simulink model "NUgus_IK"  (R2018a)
settings: Solver=VariableStepAuto  StartTime=0.0  StopTime=inf  RelTol=1e-3
values from neighbouring files (symbols this model uses):
  CM740_acc_bias = 4 * 9.80743    (= 39.22972)    [CM740_init.m]
  CM740_acc_gain = 512 / CM740_acc_centre    [CM740_init.m]
  CM740_gyro_bias = 1600 / 360 * 2 * pi    (= 27.9252680319)    [CM740_init.m]
  CM740_gyro_gain = 512 / CM740_gyro_centre    [CM740_init.m]
  head = [-0.05482228998067195, -0.00010888238321339966, 0.0011712900228573724, 0.41900000000000004]    [comtest.m]
  s = mean(abs(present_speed.data))    [RunServoTest.m]
  torso = [0.0050079703254699804, 0.008880921777563762, 0.1021503146237477, 2.5390000000000006]    [comtest.m]
undefined symbols (not defined in the file or in its folder): floor, X, Y, Z
libraries: sm_lib x211, fl_lib x128, nesl_utility x68
(part 7 of 8)

== system NUgus_IK/NUgus/right_foot/foot_bl_contact ==
  6-DOF Joint : sm_lib/Joints/6-DOF Joint  SenseConstraintForce=off  SenseConstraintForceX=off  SenseConstraintForceY=off  SenseConstraintForceZ=off  SenseConstraintTorque=off  SenseConstraintTorqueX=off  SenseConstraintTorqueY=off  SenseConstraintTorqueZ=off  SenseTotalForce=off  SenseTotalForceX=off  SenseTotalForceY=off  SenseTotalForceZ=off  SenseTotalTorque=off  SenseTotalTorqueX=off  SenseTotalTorqueY=off  SenseTotalTorqueZ=off  CompositeWrenchDir=FollowerOnBase  CompositeWrenchFrame=BaseFrame  PxEquilibriumPosition=0  PxEquilibriumPositionUnits=m  PxSpringStiffness=0  PxSpringStiffnessUnits=N/m  PxDampingCoefficient=0  PxDampingCoefficientUnits=N/(m/s)  PxTorqueActuationMode=InputTorque  PxMotionActuationMode=ComputedMotion  PxSensePosition=off  PxSenseVelocity=on  PxSenseAcceleration=off  PxSenseTorqueForce=off  PxPositionTargetSpecify=off  PxPositionTargetPriority=High  PxPositionTargetValue=0  PxPositionTargetValueUnits=m  PxVelocityTargetSpecify=off  PxVelocityTargetPriority=High  PxVelocityTargetValue=0  PxVelocityTargetValueUnits=m/s  PyEquilibriumPosition=0  PyEquilibriumPositionUnits=m  PySpringStiffness=0  PySpringStiffnessUnits=N/m  PyDampingCoefficient=0  PyDampingCoefficientUnits=N/(m/s)  PyTorqueActuationMode=InputTorque  PyMotionActuationMode=ComputedMotion  PySensePosition=off  PySenseVelocity=on  PySenseAcceleration=off  PySenseTorqueForce=off  PyPositionTargetSpecify=off  PyPositionTargetPriority=High  PyPositionTargetValue=0  PyPositionTargetValueUnits=m  PyVelocityTargetSpecify=off  PyVelocityTargetPriority=High  PyVelocityTargetValue=0  PyVelocityTargetValueUnits=m/s  PzEquilibriumPosition=0  PzEquilibriumPositionUnits=m  PzSpringStiffness=0  PzSpringStiffnessUnits=N/m  PzDampingCoefficient=0  PzDampingCoefficientUnits=N/(m/s)  PzTorqueActuationMode=InputTorque  PzMotionActuationMode=ComputedMotion  PzSensePosition=on  PzSenseVelocity=on  PzSenseAcceleration=off  PzSenseTorqueForce=off  PzPositionTargetSpecify=off  PzPositionTargetPriority=High  PzPositionTargetValue=0  PzPositionTargetValueUnits=m  PzVelocityTargetSpecify=off  PzVelocityTargetPriority=High  PzVelocityTargetValue=0  PzVelocityTargetValueUnits=m/s  SphDefPosRotationMethod=None  SphDefPosRotationAngleUnits=deg  SphDefPosRotationStandardAxis=+Z  SphDefPosRotationAngle=0.0  SphDefPosRotationArbitraryAxis=[0 0 1]  SphDefPosFollAlignAxisA=+X  SphDefPosBaseAlignAxisA=+Y  SphDefPosFollAlignAxisB=+Y  SphDefPosBaseAlignAxisB=+Z  SphDefPosRotationSequenceAxes=FollowerAxes  SphDefPosRotationSequence=XYX  SphDefPosRotationSequenceAngles=[0 0 0]  SphDefPosRotationSequenceAnglesUnits=deg  SphDefPosRotationMatrix=[1 0 0; 0 1 0; 0 0 1]  SphEqPosRotationMethod=None  SphEqPosRotationAngleUnits=deg  SphEqPosRotationStandardAxis=+Z  SphEqPosRotationAngle=0.0  SphEqPosRotationArbitraryAxis=[0 0 1]  SphEqPosFollAlignAxisA=+X  SphEqPosBaseAlignAxisA=+Y  SphEqPosFollAlignAxisB=+Y  SphEqPosBaseAlignAxisB=+Z  SphEqPosRotationSequenceAxes=FollowerAxes  SphEqPosRotationSequence=XYX  SphEqPosRotationSequenceAngles=[0 0 0]  SphEqPosRotationSequenceAnglesUnits=deg  SphEqPosRotationMatrix=[1 0 0; 0 1 0; 0 0 1]  SphSpringStiffness=0  SphSpringStiffnessUnits=N*m/deg  SphDampingCoefficient=0  SphDampingCoefficientUnits=N*m/(deg/s)  SphActuateTorqueX=off  SphActuateTorqueY=off  SphActuateTorqueZ=off  SphActuateTorque=off  SphTorqueActuationMode=NoTorque  SphMotionActuationMode=ComputedMotion  SphActuationFrame=BaseFrame  SphSensePosition=off  SphSenseVelocityX=off  SphSenseVelocityY=off  SphSenseVelocityZ=off  SphSenseVelocity=off  SphSenseAccelerationX=off  SphSenseAccelerationY=off  SphSenseAccelerationZ=off  SphSenseAcceleration=off  SphSenseTorqueX=off  SphSenseTorqueY=off  SphSenseTorqueZ=off  SphSenseTorqueForce=off  SphSensingFrame=BaseFrame  SphPositionTargetRotationMethod=None  SphPositionTargetRotationAngleUnits=deg  SphPositionTargetRotationStandardAxis=+Z  SphPositionTargetRotationAngle=0.0  SphPositionTargetRotationArbitraryAxis=[0 0 1]  SphPositionTargetFollAlignAxisA=+X  SphPositionTargetBaseAlignAxisA=+Y  SphPositionTargetFollAlignAxisB=+Y  SphPositionTargetBaseAlignAxisB=+Z  SphPositionTargetRotationSequenceAxes=FollowerAxes  SphPositionTargetRotationSequence=XYX  SphPositionTargetRotationSequenceAngles=[0 0 0]  SphPositionTargetRotationSequenceAnglesUnits=deg  SphPositionTargetRotationMatrix=[1 0 0; 0 1 0; 0 0 1]  SphPositionTargetSpecify=off  SphPositionTargetPriority=High  SphVelocityTargetValue=[0 0 0]  SphVelocityTargetValueUnits=deg/s  SphVelocityTargetSpecify=off  SphVelocityTargetPriority=High  SphVelocityTargetInFollowerFrame=on
  PS Abs1 : fl_lib/Physical Signals/Nonlinear Operators/PS Abs
      settings: SourceProductName=Simscape  SourceProductBaseCode=SS
  PS Add : fl_lib/Physical Signals/Functions/PS Add
  PS Gain : fl_lib/Physical Signals/Functions/PS Gain  gain=floor.friction
  calculate forces : Subsystem
  x Velocity Gain : fl_lib/Physical Signals/Functions/PS Gain  gain=floor.vel_gain
  y Velocity Gain : fl_lib/Physical Signals/Functions/PS Gain  gain=floor.vel_gain
  z Position Gain : fl_lib/Physical Signals/Functions/PS Gain  gain=floor.pos_gain
  z Velocity Gain : fl_lib/Physical Signals/Functions/PS Gain  gain=floor.vel_gain
  Contact : PMIOPort  Side=Right
  Floor : PMIOPort  Port=2  Side=Left
  connections:
  6-DOF Joint/RConn1 -- Contact/RConn1
  Floor/RConn1 -- 6-DOF Joint/LConn1
  6-DOF Joint/RConn4 -- calculate forces/LConn3 -- z Position Gain/LConn1
  z Velocity Gain/LConn1 -- 6-DOF Joint/RConn5
  y Velocity Gain/LConn1 -- 6-DOF Joint/RConn3
  x Velocity Gain/LConn1 -- 6-DOF Joint/RConn2
  PS Add/LConn1 -- z Position Gain/RConn1
  PS Add/LConn2 -- z Velocity Gain/RConn1
  PS Abs1/LConn1 -- PS Gain/RConn1
  PS Add/RConn1 -- calculate forces/LConn4 -- PS Gain/LConn1
  x Velocity Gain/RConn1 -- calculate forces/LConn1
  y Velocity Gain/RConn1 -- calculate forces/LConn2
  PS Abs1/RConn1 -- calculate forces/LConn5
  calculate forces/RConn1 -- 6-DOF Joint/LConn2
  calculate forces/RConn2 -- 6-DOF Joint/LConn3
  calculate forces/RConn3 -- 6-DOF Joint/LConn4

== system NUgus_IK/NUgus/right_foot/foot_br_contact ==
  6-DOF Joint : sm_lib/Joints/6-DOF Joint  SenseConstraintForce=off  SenseConstraintForceX=off  SenseConstraintForceY=off  SenseConstraintForceZ=off  SenseConstraintTorque=off  SenseConstraintTorqueX=off  SenseConstraintTorqueY=off  SenseConstraintTorqueZ=off  SenseTotalForce=off  SenseTotalForceX=off  SenseTotalForceY=off  SenseTotalForceZ=off  SenseTotalTorque=off  SenseTotalTorqueX=off  SenseTotalTorqueY=off  SenseTotalTorqueZ=off  CompositeWrenchDir=FollowerOnBase  CompositeWrenchFrame=BaseFrame  PxEquilibriumPosition=0  PxEquilibriumPositionUnits=m  PxSpringStiffness=0  PxSpringStiffnessUnits=N/m  PxDampingCoefficient=0  PxDampingCoefficientUnits=N/(m/s)  PxTorqueActuationMode=InputTorque  PxMotionActuationMode=ComputedMotion  PxSensePosition=off  PxSenseVelocity=on  PxSenseAcceleration=off  PxSenseTorqueForce=off  PxPositionTargetSpecify=off  PxPositionTargetPriority=High  PxPositionTargetValue=0  PxPositionTargetValueUnits=m  PxVelocityTargetSpecify=off  PxVelocityTargetPriority=High  PxVelocityTargetValue=0  PxVelocityTargetValueUnits=m/s  PyEquilibriumPosition=0  PyEquilibriumPositionUnits=m  PySpringStiffness=0  PySpringStiffnessUnits=N/m  PyDampingCoefficient=0  PyDampingCoefficientUnits=N/(m/s)  PyTorqueActuationMode=InputTorque  PyMotionActuationMode=ComputedMotion  PySensePosition=off  PySenseVelocity=on  PySenseAcceleration=off  PySenseTorqueForce=off  PyPositionTargetSpecify=off  PyPositionTargetPriority=High  PyPositionTargetValue=0  PyPositionTargetValueUnits=m  PyVelocityTargetSpecify=off  PyVelocityTargetPriority=High  PyVelocityTargetValue=0  PyVelocityTargetValueUnits=m/s  PzEquilibriumPosition=0  PzEquilibriumPositionUnits=m  PzSpringStiffness=0  PzSpringStiffnessUnits=N/m  PzDampingCoefficient=0  PzDampingCoefficientUnits=N/(m/s)  PzTorqueActuationMode=InputTorque  PzMotionActuationMode=ComputedMotion  PzSensePosition=on  PzSenseVelocity=on  PzSenseAcceleration=off  PzSenseTorqueForce=off  PzPositionTargetSpecify=off  PzPositionTargetPriority=High  PzPositionTargetValue=0  PzPositionTargetValueUnits=m  PzVelocityTargetSpecify=off  PzVelocityTargetPriority=High  PzVelocityTargetValue=0  PzVelocityTargetValueUnits=m/s  SphDefPosRotationMethod=None  SphDefPosRotationAngleUnits=deg  SphDefPosRotationStandardAxis=+Z  SphDefPosRotationAngle=0.0  SphDefPosRotationArbitraryAxis=[0 0 1]  SphDefPosFollAlignAxisA=+X  SphDefPosBaseAlignAxisA=+Y  SphDefPosFollAlignAxisB=+Y  SphDefPosBaseAlignAxisB=+Z  SphDefPosRotationSequenceAxes=FollowerAxes  SphDefPosRotationSequence=XYX  SphDefPosRotationSequenceAngles=[0 0 0]  SphDefPosRotationSequenceAnglesUnits=deg  SphDefPosRotationMatrix=[1 0 0; 0 1 0; 0 0 1]  SphEqPosRotationMethod=None  SphEqPosRotationAngleUnits=deg  SphEqPosRotationStandardAxis=+Z  SphEqPosRotationAngle=0.0  SphEqPosRotationArbitraryAxis=[0 0 1]  SphEqPosFollAlignAxisA=+X  SphEqPosBaseAlignAxisA=+Y  SphEqPosFollAlignAxisB=+Y  SphEqPosBaseAlignAxisB=+Z  SphEqPosRotationSequenceAxes=FollowerAxes  SphEqPosRotationSequence=XYX  SphEqPosRotationSequenceAngles=[0 0 0]  SphEqPosRotationSequenceAnglesUnits=deg  SphEqPosRotationMatrix=[1 0 0; 0 1 0; 0 0 1]  SphSpringStiffness=0  SphSpringStiffnessUnits=N*m/deg  SphDampingCoefficient=0  SphDampingCoefficientUnits=N*m/(deg/s)  SphActuateTorqueX=off  SphActuateTorqueY=off  SphActuateTorqueZ=off  SphActuateTorque=off  SphTorqueActuationMode=NoTorque  SphMotionActuationMode=ComputedMotion  SphActuationFrame=BaseFrame  SphSensePosition=off  SphSenseVelocityX=off  SphSenseVelocityY=off  SphSenseVelocityZ=off  SphSenseVelocity=off  SphSenseAccelerationX=off  SphSenseAccelerationY=off  SphSenseAccelerationZ=off  SphSenseAcceleration=off  SphSenseTorqueX=off  SphSenseTorqueY=off  SphSenseTorqueZ=off  SphSenseTorqueForce=off  SphSensingFrame=BaseFrame  SphPositionTargetRotationMethod=None  SphPositionTargetRotationAngleUnits=deg  SphPositionTargetRotationStandardAxis=+Z  SphPositionTargetRotationAngle=0.0  SphPositionTargetRotationArbitraryAxis=[0 0 1]  SphPositionTargetFollAlignAxisA=+X  SphPositionTargetBaseAlignAxisA=+Y  SphPositionTargetFollAlignAxisB=+Y  SphPositionTargetBaseAlignAxisB=+Z  SphPositionTargetRotationSequenceAxes=FollowerAxes  SphPositionTargetRotationSequence=XYX  SphPositionTargetRotationSequenceAngles=[0 0 0]  SphPositionTargetRotationSequenceAnglesUnits=deg  SphPositionTargetRotationMatrix=[1 0 0; 0 1 0; 0 0 1]  SphPositionTargetSpecify=off  SphPositionTargetPriority=High  SphVelocityTargetValue=[0 0 0]  SphVelocityTargetValueUnits=deg/s  SphVelocityTargetSpecify=off  SphVelocityTargetPriority=High  SphVelocityTargetInFollowerFrame=on
  PS Abs1 : fl_lib/Physical Signals/Nonlinear Operators/PS Abs
      settings: SourceProductName=Simscape  SourceProductBaseCode=SS
  PS Add : fl_lib/Physical Signals/Functions/PS Add
  PS Gain : fl_lib/Physical Signals/Functions/PS Gain  gain=floor.friction
  calculate forces : Subsystem
  x Velocity Gain : fl_lib/Physical Signals/Functions/PS Gain  gain=floor.vel_gain
  y Velocity Gain : fl_lib/Physical Signals/Functions/PS Gain  gain=floor.vel_gain
  z Position Gain : fl_lib/Physical Signals/Functions/PS Gain  gain=floor.pos_gain
  z Velocity Gain : fl_lib/Physical Signals/Functions/PS Gain  gain=floor.vel_gain
  Contact : PMIOPort  Side=Right
  Floor : PMIOPort  Port=2  Side=Left
  connections:
  6-DOF Joint/RConn1 -- Contact/RConn1
  Floor/RConn1 -- 6-DOF Joint/LConn1
  6-DOF Joint/RConn4 -- calculate forces/LConn3 -- z Position Gain/LConn1
  z Velocity Gain/LConn1 -- 6-DOF Joint/RConn5
  y Velocity Gain/LConn1 -- 6-DOF Joint/RConn3
  x Velocity Gain/LConn1 -- 6-DOF Joint/RConn2
  PS Add/LConn1 -- z Position Gain/RConn1
  PS Add/LConn2 -- z Velocity Gain/RConn1
  PS Abs1/LConn1 -- PS Gain/RConn1
  PS Add/RConn1 -- calculate forces/LConn4 -- PS Gain/LConn1
  x Velocity Gain/RConn1 -- calculate forces/LConn1
  y Velocity Gain/RConn1 -- calculate forces/LConn2
  PS Abs1/RConn1 -- calculate forces/LConn5
  calculate forces/RConn1 -- 6-DOF Joint/LConn2
  calculate forces/RConn2 -- 6-DOF Joint/LConn3
  calculate forces/RConn3 -- 6-DOF Joint/LConn4

== system NUgus_IK/NUgus/right_foot/foot_fl_contact ==
  6-DOF Joint : sm_lib/Joints/6-DOF Joint  SenseConstraintForce=off  SenseConstraintForceX=off  SenseConstraintForceY=off  SenseConstraintForceZ=off  SenseConstraintTorque=off  SenseConstraintTorqueX=off  SenseConstraintTorqueY=off  SenseConstraintTorqueZ=off  SenseTotalForce=off  SenseTotalForceX=off  SenseTotalForceY=off  SenseTotalForceZ=off  SenseTotalTorque=off  SenseTotalTorqueX=off  SenseTotalTorqueY=off  SenseTotalTorqueZ=off  CompositeWrenchDir=FollowerOnBase  CompositeWrenchFrame=BaseFrame  PxEquilibriumPosition=0  PxEquilibriumPositionUnits=m  PxSpringStiffness=0  PxSpringStiffnessUnits=N/m  PxDampingCoefficient=0  PxDampingCoefficientUnits=N/(m/s)  PxTorqueActuationMode=InputTorque  PxMotionActuationMode=ComputedMotion  PxSensePosition=off  PxSenseVelocity=on  PxSenseAcceleration=off  PxSenseTorqueForce=off  PxPositionTargetSpecify=off  PxPositionTargetPriority=High  PxPositionTargetValue=0  PxPositionTargetValueUnits=m  PxVelocityTargetSpecify=off  PxVelocityTargetPriority=High  PxVelocityTargetValue=0  PxVelocityTargetValueUnits=m/s  PyEquilibriumPosition=0  PyEquilibriumPositionUnits=m  PySpringStiffness=0  PySpringStiffnessUnits=N/m  PyDampingCoefficient=0  PyDampingCoefficientUnits=N/(m/s)  PyTorqueActuationMode=InputTorque  PyMotionActuationMode=ComputedMotion  PySensePosition=off  PySenseVelocity=on  PySenseAcceleration=off  PySenseTorqueForce=off  PyPositionTargetSpecify=off  PyPositionTargetPriority=High  PyPositionTargetValue=0  PyPositionTargetValueUnits=m  PyVelocityTargetSpecify=off  PyVelocityTargetPriority=High  PyVelocityTargetValue=0  PyVelocityTargetValueUnits=m/s  PzEquilibriumPosition=0  PzEquilibriumPositionUnits=m  PzSpringStiffness=0  PzSpringStiffnessUnits=N/m  PzDampingCoefficient=0  PzDampingCoefficientUnits=N/(m/s)  PzTorqueActuationMode=InputTorque  PzMotionActuationMode=ComputedMotion  PzSensePosition=on  PzSenseVelocity=on  PzSenseAcceleration=off  PzSenseTorqueForce=off  PzPositionTargetSpecify=off  PzPositionTargetPriority=High  PzPositionTargetValue=0  PzPositionTargetValueUnits=m  PzVelocityTargetSpecify=off  PzVelocityTargetPriority=High  PzVelocityTargetValue=0  PzVelocityTargetValueUnits=m/s  SphDefPosRotationMethod=None  SphDefPosRotationAngleUnits=deg  SphDefPosRotationStandardAxis=+Z  SphDefPosRotationAngle=0.0  SphDefPosRotationArbitraryAxis=[0 0 1]  SphDefPosFollAlignAxisA=+X  SphDefPosBaseAlignAxisA=+Y  SphDefPosFollAlignAxisB=+Y  SphDefPosBaseAlignAxisB=+Z  SphDefPosRotationSequenceAxes=FollowerAxes  SphDefPosRotationSequence=XYX  SphDefPosRotationSequenceAngles=[0 0 0]  SphDefPosRotationSequenceAnglesUnits=deg  SphDefPosRotationMatrix=[1 0 0; 0 1 0; 0 0 1]  SphEqPosRotationMethod=None  SphEqPosRotationAngleUnits=deg  SphEqPosRotationStandardAxis=+Z  SphEqPosRotationAngle=0.0  SphEqPosRotationArbitraryAxis=[0 0 1]  SphEqPosFollAlignAxisA=+X  SphEqPosBaseAlignAxisA=+Y  SphEqPosFollAlignAxisB=+Y  SphEqPosBaseAlignAxisB=+Z  SphEqPosRotationSequenceAxes=FollowerAxes  SphEqPosRotationSequence=XYX  SphEqPosRotationSequenceAngles=[0 0 0]  SphEqPosRotationSequenceAnglesUnits=deg  SphEqPosRotationMatrix=[1 0 0; 0 1 0; 0 0 1]  SphSpringStiffness=0  SphSpringStiffnessUnits=N*m/deg  SphDampingCoefficient=0  SphDampingCoefficientUnits=N*m/(deg/s)  SphActuateTorqueX=off  SphActuateTorqueY=off  SphActuateTorqueZ=off  SphActuateTorque=off  SphTorqueActuationMode=NoTorque  SphMotionActuationMode=ComputedMotion  SphActuationFrame=BaseFrame  SphSensePosition=off  SphSenseVelocityX=off  SphSenseVelocityY=off  SphSenseVelocityZ=off  SphSenseVelocity=off  SphSenseAccelerationX=off  SphSenseAccelerationY=off  SphSenseAccelerationZ=off  SphSenseAcceleration=off  SphSenseTorqueX=off  SphSenseTorqueY=off  SphSenseTorqueZ=off  SphSenseTorqueForce=off  SphSensingFrame=BaseFrame  SphPositionTargetRotationMethod=None  SphPositionTargetRotationAngleUnits=deg  SphPositionTargetRotationStandardAxis=+Z  SphPositionTargetRotationAngle=0.0  SphPositionTargetRotationArbitraryAxis=[0 0 1]  SphPositionTargetFollAlignAxisA=+X  SphPositionTargetBaseAlignAxisA=+Y  SphPositionTargetFollAlignAxisB=+Y  SphPositionTargetBaseAlignAxisB=+Z  SphPositionTargetRotationSequenceAxes=FollowerAxes  SphPositionTargetRotationSequence=XYX  SphPositionTargetRotationSequenceAngles=[0 0 0]  SphPositionTargetRotationSequenceAnglesUnits=deg  SphPositionTargetRotationMatrix=[1 0 0; 0 1 0; 0 0 1]  SphPositionTargetSpecify=off  SphPositionTargetPriority=High  SphVelocityTargetValue=[0 0 0]  SphVelocityTargetValueUnits=deg/s  SphVelocityTargetSpecify=off  SphVelocityTargetPriority=High  SphVelocityTargetInFollowerFrame=on
  PS Abs1 : fl_lib/Physical Signals/Nonlinear Operators/PS Abs
      settings: SourceProductName=Simscape  SourceProductBaseCode=SS
  PS Add : fl_lib/Physical Signals/Functions/PS Add
  PS Gain : fl_lib/Physical Signals/Functions/PS Gain  gain=floor.friction
  calculate forces : Subsystem
  x Velocity Gain : fl_lib/Physical Signals/Functions/PS Gain  gain=floor.vel_gain
  y Velocity Gain : fl_lib/Physical Signals/Functions/PS Gain  gain=floor.vel_gain
  z Position Gain : fl_lib/Physical Signals/Functions/PS Gain  gain=floor.pos_gain
  z Velocity Gain : fl_lib/Physical Signals/Functions/PS Gain  gain=floor.vel_gain
  Contact : PMIOPort  Side=Right
  Floor : PMIOPort  Port=2  Side=Left
  connections:
  6-DOF Joint/RConn1 -- Contact/RConn1
  Floor/RConn1 -- 6-DOF Joint/LConn1
  6-DOF Joint/RConn4 -- calculate forces/LConn3 -- z Position Gain/LConn1
  z Velocity Gain/LConn1 -- 6-DOF Joint/RConn5
  y Velocity Gain/LConn1 -- 6-DOF Joint/RConn3
  x Velocity Gain/LConn1 -- 6-DOF Joint/RConn2
  PS Add/LConn1 -- z Position Gain/RConn1
  PS Add/LConn2 -- z Velocity Gain/RConn1
  PS Abs1/LConn1 -- PS Gain/RConn1
  PS Add/RConn1 -- calculate forces/LConn4 -- PS Gain/LConn1
  x Velocity Gain/RConn1 -- calculate forces/LConn1
  y Velocity Gain/RConn1 -- calculate forces/LConn2
  PS Abs1/RConn1 -- calculate forces/LConn5
  calculate forces/RConn1 -- 6-DOF Joint/LConn2
  calculate forces/RConn2 -- 6-DOF Joint/LConn3
  calculate forces/RConn3 -- 6-DOF Joint/LConn4

== system NUgus_IK/NUgus/right_foot/foot_fr_contact ==
  6-DOF Joint : sm_lib/Joints/6-DOF Joint  SenseConstraintForce=off  SenseConstraintForceX=off  SenseConstraintForceY=off  SenseConstraintForceZ=off  SenseConstraintTorque=off  SenseConstraintTorqueX=off  SenseConstraintTorqueY=off  SenseConstraintTorqueZ=off  SenseTotalForce=off  SenseTotalForceX=off  SenseTotalForceY=off  SenseTotalForceZ=off  SenseTotalTorque=off  SenseTotalTorqueX=off  SenseTotalTorqueY=off  SenseTotalTorqueZ=off  CompositeWrenchDir=FollowerOnBase  CompositeWrenchFrame=BaseFrame  PxEquilibriumPosition=0  PxEquilibriumPositionUnits=m  PxSpringStiffness=0  PxSpringStiffnessUnits=N/m  PxDampingCoefficient=0  PxDampingCoefficientUnits=N/(m/s)  PxTorqueActuationMode=InputTorque  PxMotionActuationMode=ComputedMotion  PxSensePosition=off  PxSenseVelocity=on  PxSenseAcceleration=off  PxSenseTorqueForce=off  PxPositionTargetSpecify=off  PxPositionTargetPriority=High  PxPositionTargetValue=0  PxPositionTargetValueUnits=m  PxVelocityTargetSpecify=off  PxVelocityTargetPriority=High  PxVelocityTargetValue=0  PxVelocityTargetValueUnits=m/s  PyEquilibriumPosition=0  PyEquilibriumPositionUnits=m  PySpringStiffness=0  PySpringStiffnessUnits=N/m  PyDampingCoefficient=0  PyDampingCoefficientUnits=N/(m/s)  PyTorqueActuationMode=InputTorque  PyMotionActuationMode=ComputedMotion  PySensePosition=off  PySenseVelocity=on  PySenseAcceleration=off  PySenseTorqueForce=off  PyPositionTargetSpecify=off  PyPositionTargetPriority=High  PyPositionTargetValue=0  PyPositionTargetValueUnits=m  PyVelocityTargetSpecify=off  PyVelocityTargetPriority=High  PyVelocityTargetValue=0  PyVelocityTargetValueUnits=m/s  PzEquilibriumPosition=0  PzEquilibriumPositionUnits=m  PzSpringStiffness=0  PzSpringStiffnessUnits=N/m  PzDampingCoefficient=0  PzDampingCoefficientUnits=N/(m/s)  PzTorqueActuationMode=InputTorque  PzMotionActuationMode=ComputedMotion  PzSensePosition=on  PzSenseVelocity=on  PzSenseAcceleration=off  PzSenseTorqueForce=off  PzPositionTargetSpecify=off  PzPositionTargetPriority=High  PzPositionTargetValue=0  PzPositionTargetValueUnits=m  PzVelocityTargetSpecify=off  PzVelocityTargetPriority=High  PzVelocityTargetValue=0  PzVelocityTargetValueUnits=m/s  SphDefPosRotationMethod=None  SphDefPosRotationAngleUnits=deg  SphDefPosRotationStandardAxis=+Z  SphDefPosRotationAngle=0.0  SphDefPosRotationArbitraryAxis=[0 0 1]  SphDefPosFollAlignAxisA=+X  SphDefPosBaseAlignAxisA=+Y  SphDefPosFollAlignAxisB=+Y  SphDefPosBaseAlignAxisB=+Z  SphDefPosRotationSequenceAxes=FollowerAxes  SphDefPosRotationSequence=XYX  SphDefPosRotationSequenceAngles=[0 0 0]  SphDefPosRotationSequenceAnglesUnits=deg  SphDefPosRotationMatrix=[1 0 0; 0 1 0; 0 0 1]  SphEqPosRotationMethod=None  SphEqPosRotationAngleUnits=deg  SphEqPosRotationStandardAxis=+Z  SphEqPosRotationAngle=0.0  SphEqPosRotationArbitraryAxis=[0 0 1]  SphEqPosFollAlignAxisA=+X  SphEqPosBaseAlignAxisA=+Y  SphEqPosFollAlignAxisB=+Y  SphEqPosBaseAlignAxisB=+Z  SphEqPosRotationSequenceAxes=FollowerAxes  SphEqPosRotationSequence=XYX  SphEqPosRotationSequenceAngles=[0 0 0]  SphEqPosRotationSequenceAnglesUnits=deg  SphEqPosRotationMatrix=[1 0 0; 0 1 0; 0 0 1]  SphSpringStiffness=0  SphSpringStiffnessUnits=N*m/deg  SphDampingCoefficient=0  SphDampingCoefficientUnits=N*m/(deg/s)  SphActuateTorqueX=off  SphActuateTorqueY=off  SphActuateTorqueZ=off  SphActuateTorque=off  SphTorqueActuationMode=NoTorque  SphMotionActuationMode=ComputedMotion  SphActuationFrame=BaseFrame  SphSensePosition=off  SphSenseVelocityX=off  SphSenseVelocityY=off  SphSenseVelocityZ=off  SphSenseVelocity=off  SphSenseAccelerationX=off  SphSenseAccelerationY=off  SphSenseAccelerationZ=off  SphSenseAcceleration=off  SphSenseTorqueX=off  SphSenseTorqueY=off  SphSenseTorqueZ=off  SphSenseTorqueForce=off  SphSensingFrame=BaseFrame  SphPositionTargetRotationMethod=None  SphPositionTargetRotationAngleUnits=deg  SphPositionTargetRotationStandardAxis=+Z  SphPositionTargetRotationAngle=0.0  SphPositionTargetRotationArbitraryAxis=[0 0 1]  SphPositionTargetFollAlignAxisA=+X  SphPositionTargetBaseAlignAxisA=+Y  SphPositionTargetFollAlignAxisB=+Y  SphPositionTargetBaseAlignAxisB=+Z  SphPositionTargetRotationSequenceAxes=FollowerAxes  SphPositionTargetRotationSequence=XYX  SphPositionTargetRotationSequenceAngles=[0 0 0]  SphPositionTargetRotationSequenceAnglesUnits=deg  SphPositionTargetRotationMatrix=[1 0 0; 0 1 0; 0 0 1]  SphPositionTargetSpecify=off  SphPositionTargetPriority=High  SphVelocityTargetValue=[0 0 0]  SphVelocityTargetValueUnits=deg/s  SphVelocityTargetSpecify=off  SphVelocityTargetPriority=High  SphVelocityTargetInFollowerFrame=on
  PS Abs1 : fl_lib/Physical Signals/Nonlinear Operators/PS Abs
      settings: SourceProductName=Simscape  SourceProductBaseCode=SS
  PS Add : fl_lib/Physical Signals/Functions/PS Add
  PS Gain : fl_lib/Physical Signals/Functions/PS Gain  gain=floor.friction
  calculate forces : Subsystem
  x Velocity Gain : fl_lib/Physical Signals/Functions/PS Gain  gain=floor.vel_gain
  y Velocity Gain : fl_lib/Physical Signals/Functions/PS Gain  gain=floor.vel_gain
  z Position Gain : fl_lib/Physical Signals/Functions/PS Gain  gain=floor.pos_gain
  z Velocity Gain : fl_lib/Physical Signals/Functions/PS Gain  gain=floor.vel_gain
  Contact : PMIOPort  Side=Right
  Floor : PMIOPort  Port=2  Side=Left
  connections:
  6-DOF Joint/RConn1 -- Contact/RConn1
  Floor/RConn1 -- 6-DOF Joint/LConn1
  6-DOF Joint/RConn4 -- calculate forces/LConn3 -- z Position Gain/LConn1
  z Velocity Gain/LConn1 -- 6-DOF Joint/RConn5
  y Velocity Gain/LConn1 -- 6-DOF Joint/RConn3
  x Velocity Gain/LConn1 -- 6-DOF Joint/RConn2
  PS Add/LConn1 -- z Position Gain/RConn1
  PS Add/LConn2 -- z Velocity Gain/RConn1
  PS Abs1/LConn1 -- PS Gain/RConn1
  PS Add/RConn1 -- calculate forces/LConn4 -- PS Gain/LConn1
  x Velocity Gain/RConn1 -- calculate forces/LConn1
  y Velocity Gain/RConn1 -- calculate forces/LConn2
  PS Abs1/RConn1 -- calculate forces/LConn5
  calculate forces/RConn1 -- 6-DOF Joint/LConn2
  calculate forces/RConn2 -- 6-DOF Joint/LConn3
  calculate forces/RConn3 -- 6-DOF Joint/LConn4

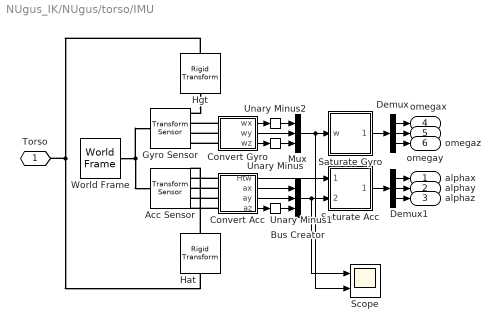
== system NUgus_IK/NUgus/torso/IMU ==
  Acc Sensor : sm_lib/Frames and Transforms/Transform Sensor  MeasurementFrame=Follower  SenseAngle=off  SenseAxis=off  SenseAngle1=off  SenseAngle2=off  SenseAngle3=off  SenseQ=off  SenseR=on  SenseOmegaX=off  SenseOmegaY=off  SenseOmegaZ=off  SenseOmega1=off  SenseOmega2=off  SenseOmega3=off  SenseQDot=off  SenseRDot=off  SenseAlphaX=off  SenseAlphaY=off  SenseAlphaZ=off  SenseAlpha1=off  SenseAlpha2=off  SenseAlpha3=off  SenseQDDot=off  SenseRDDot=off  SenseX=off  SenseY=off  SenseZ=off  SenseRad=off  SenseAzim=off  SenseDist=off  SenseInc=off  SenseXDot=off  SenseYDot=off  SenseZDot=off  SenseRadDot=off  SenseAzimDot=off  SenseDistDot=off  SenseIncDot=off  SenseXDDot=on  SenseYDDot=on  SenseZDDot=on  SenseRadDDot=off  SenseAzimDDot=off  SenseDistDDot=off  SenseIncDDot=off
  Bus Creator : BusCreator  Inputs=3
  Convert Acc : Subsystem
  Convert Gyro : Subsystem
  Demux : Demux  Outputs=3
  Demux1 : Demux  Outputs=3
  Gyro Sensor : sm_lib/Frames and Transforms/Transform Sensor  MeasurementFrame=Follower  SenseAngle=off  SenseAxis=off  SenseAngle1=off  SenseAngle2=off  SenseAngle3=off  SenseQ=off  SenseR=off  SenseOmegaX=on  SenseOmegaY=on  SenseOmegaZ=on  SenseOmega1=off  SenseOmega2=off  SenseOmega3=off  SenseQDot=off  SenseRDot=off  SenseAlphaX=off  SenseAlphaY=off  SenseAlphaZ=off  SenseAlpha1=off  SenseAlpha2=off  SenseAlpha3=off  SenseQDDot=off  SenseRDDot=off  SenseX=off  SenseY=off  SenseZ=off  SenseRad=off  SenseAzim=off  SenseDist=off  SenseInc=off  SenseXDot=off  SenseYDot=off  SenseZDot=off  SenseRadDot=off  SenseAzimDot=off  SenseDistDot=off  SenseIncDot=off  SenseXDDot=off  SenseYDDot=off  SenseZDDot=off  SenseRadDDot=off  SenseAzimDDot=off  SenseDistDDot=off  SenseIncDDot=off
  Hat : sm_lib/Frames and Transforms/Rigid Transform  TranslationMethod=None  TranslationStandardOffset=0  TranslationLengthUnit=m  TranslationStandardAxis=+Z  TranslationCartesianOffset=[0 0 0]  TranslationROffset=0  TranslationROffsetUnits=m  TranslationZOffset=0  TranslationZOffsetUnits=m  TranslationThetaOffset=0  TranslationThetaOffsetUnits=deg  RotationMethod=None  RotationAngleUnits=deg  RotationStandardAxis=+Z  RotationAngle=0.0  RotationArbitraryAxis=[0 0 1]  FollAlignAxisA=+X  BaseAlignAxisA=+Y  FollAlignAxisB=+Y  BaseAlignAxisB=+Z  RotationSequenceAxes=FollowerAxes  RotationSequence=XYX  RotationSequenceAngles=[0 0 0]  RotationSequenceAnglesUnits=deg  RotationMatrix=[1 0 0; 0 1 0; 0 0 1]
  Hgt : sm_lib/Frames and Transforms/Rigid Transform  TranslationMethod=None  TranslationStandardOffset=0  TranslationLengthUnit=m  TranslationStandardAxis=+Z  TranslationCartesianOffset=[0 0 0]  TranslationROffset=0  TranslationROffsetUnits=m  TranslationZOffset=0  TranslationZOffsetUnits=m  TranslationThetaOffset=0  TranslationThetaOffsetUnits=deg  RotationMethod=None  RotationAngleUnits=deg  RotationStandardAxis=+Z  RotationAngle=0.0  RotationArbitraryAxis=[0 0 1]  FollAlignAxisA=+X  BaseAlignAxisA=+Y  FollAlignAxisB=+Y  BaseAlignAxisB=+Z  RotationSequenceAxes=FollowerAxes  RotationSequence=XYX  RotationSequenceAngles=[0 0 0]  RotationSequenceAnglesUnits=deg  RotationMatrix=[1 0 0; 0 1 0; 0 0 1]
  Mux : Mux  Inputs=3
  Saturate Acc : Subsystem
  Saturate Gyro : Subsystem
  Scope : Scope  NumInputPorts=2
  Unary Minus : UnaryMinus
  Unary Minus1 : UnaryMinus
  Unary Minus2 : UnaryMinus
  World Frame : sm_lib/Frames and Transforms/World Frame
  Torso : PMIOPort  Side=Left
  alphax : Outport
  alphay : Outport  Port=2
  alphaz : Outport  Port=3
  omegax : Outport  Port=4
  omegay : Outport  Port=5
  omegaz : Outport  Port=6
  wires:
  Convert Acc/3(ay) -> Bus Creator/2
  Convert Gyro/2(wy) -> Mux/2
  Convert Gyro/3(wz) -> Unary Minus/1
  Unary Minus/1 -> Mux/3
  Convert Gyro/1(wx) -> Unary Minus2/1
  Unary Minus2/1 -> Mux/1
  Convert Acc/2(ax) -> Bus Creator/1
  Unary Minus1/1 -> Bus Creator/3
  Demux/1 -> omegax/1
  Demux/2 -> omegay/1
  Demux/3 -> omegaz/1
  Demux1/3 -> alphaz/1
  Demux1/1 -> alphax/1
  Demux1/2 -> alphay/1
  Saturate Acc/1(alpha) -> Demux1/1
  Convert Acc/4(az) -> Unary Minus1/1
  Convert Acc/1(Htw) -> Saturate Acc/1(Hta)
  Bus Creator/1 -> Scope/1, Saturate Acc/2(Acc)
  Mux/1 -> Scope/2, Saturate Gyro/1(w)
  Saturate Gyro/1(omega) -> Demux/1
  connections:
  Convert Acc/LConn4 -- Acc Sensor/RConn5
  Convert Gyro/LConn2 -- Gyro Sensor/RConn3
  Convert Acc/LConn3 -- Acc Sensor/RConn4
  Hgt/LConn1 -- Hat/LConn1 -- Torso/RConn1
  Convert Gyro/LConn3 -- Gyro Sensor/RConn4
  Convert Acc/LConn2 -- Acc Sensor/RConn3
  Convert Gyro/LConn1 -- Gyro Sensor/RConn2
  World Frame/RConn1 -- Gyro Sensor/LConn1 -- Acc Sensor/LConn1
  Hat/RConn1 -- Acc Sensor/RConn1
  Convert Acc/LConn1 -- Acc Sensor/RConn2
  Hgt/RConn1 -- Gyro Sensor/RConn1

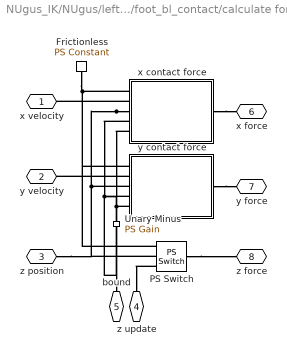
== system NUgus_IK/NUgus/left_foot/foot_bl_contact/calculate forces ==
  Frictionless : fl_lib/Physical Signals/Sources/PS Constant  constant=0
  PS Switch : fl_lib/Physical Signals/Nonlinear Operators/PS Switch  Threshold=0
      settings: SourceProductName=Simscape  SourceProductBaseCode=SS
  Unary Minus : fl_lib/Physical Signals/Functions/PS Gain  gain=-1
  x contact force : Subsystem
  y contact force : Subsystem
  x velocity : PMIOPort  Side=Left
  y velocity : PMIOPort  Port=2  Side=Left
  z position : PMIOPort  Port=3  Side=Left
  z update : PMIOPort  Port=4  Side=Left
  bound : PMIOPort  Port=5  Side=Left
  x force : PMIOPort  Port=6  Side=Right
  y force : PMIOPort  Port=7  Side=Right
  z force : PMIOPort  Port=8  Side=Right
  connections:
  x contact force/LConn2 -- x velocity/RConn1
  y contact force/LConn2 -- y velocity/RConn1
  y contact force/RConn1 -- y force/RConn1
  x contact force/RConn1 -- x force/RConn1
  PS Switch/RConn1 -- z force/RConn1
  x contact force/LConn3 -- PS Switch/LConn2 -- z position/RConn1 -- y contact force/LConn3
  x contact force/LConn4 -- Unary Minus/LConn1 -- bound/RConn1 -- y contact force/LConn4
  Unary Minus/RConn1 -- x contact force/LConn5 -- y contact force/LConn5
  x contact force/LConn1 -- y contact force/LConn1 -- PS Switch/LConn1 -- Frictionless/RConn1
  PS Switch/LConn3 -- z update/RConn1

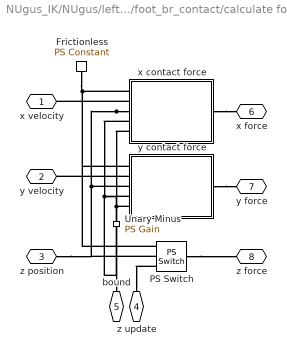
== system NUgus_IK/NUgus/left_foot/foot_br_contact/calculate forces ==
  Frictionless : fl_lib/Physical Signals/Sources/PS Constant  constant=0
  PS Switch : fl_lib/Physical Signals/Nonlinear Operators/PS Switch  Threshold=0
      settings: SourceProductName=Simscape  SourceProductBaseCode=SS
  Unary Minus : fl_lib/Physical Signals/Functions/PS Gain  gain=-1
  x contact force : Subsystem
  y contact force : Subsystem
  x velocity : PMIOPort  Side=Left
  y velocity : PMIOPort  Port=2  Side=Left
  z position : PMIOPort  Port=3  Side=Left
  z update : PMIOPort  Port=4  Side=Left
  bound : PMIOPort  Port=5  Side=Left
  x force : PMIOPort  Port=6  Side=Right
  y force : PMIOPort  Port=7  Side=Right
  z force : PMIOPort  Port=8  Side=Right
  connections:
  x contact force/LConn2 -- x velocity/RConn1
  y contact force/LConn2 -- y velocity/RConn1
  y contact force/RConn1 -- y force/RConn1
  x contact force/RConn1 -- x force/RConn1
  PS Switch/RConn1 -- z force/RConn1
  x contact force/LConn3 -- PS Switch/LConn2 -- z position/RConn1 -- y contact force/LConn3
  x contact force/LConn4 -- Unary Minus/LConn1 -- bound/RConn1 -- y contact force/LConn4
  Unary Minus/RConn1 -- x contact force/LConn5 -- y contact force/LConn5
  x contact force/LConn1 -- y contact force/LConn1 -- PS Switch/LConn1 -- Frictionless/RConn1
  PS Switch/LConn3 -- z update/RConn1

== system NUgus_IK/NUgus/left_foot/foot_fl_contact/calculate forces ==
  Frictionless : fl_lib/Physical Signals/Sources/PS Constant  constant=0
  PS Switch : fl_lib/Physical Signals/Nonlinear Operators/PS Switch  Threshold=0
      settings: SourceProductName=Simscape  SourceProductBaseCode=SS
  Unary Minus : fl_lib/Physical Signals/Functions/PS Gain  gain=-1
  x contact force : Subsystem
  y contact force : Subsystem
  x velocity : PMIOPort  Side=Left
  y velocity : PMIOPort  Port=2  Side=Left
  z position : PMIOPort  Port=3  Side=Left
  z update : PMIOPort  Port=4  Side=Left
  bound : PMIOPort  Port=5  Side=Left
  x force : PMIOPort  Port=6  Side=Right
  y force : PMIOPort  Port=7  Side=Right
  z force : PMIOPort  Port=8  Side=Right
  connections:
  x contact force/LConn2 -- x velocity/RConn1
  y contact force/LConn2 -- y velocity/RConn1
  y contact force/RConn1 -- y force/RConn1
  x contact force/RConn1 -- x force/RConn1
  PS Switch/RConn1 -- z force/RConn1
  x contact force/LConn3 -- PS Switch/LConn2 -- z position/RConn1 -- y contact force/LConn3
  x contact force/LConn4 -- Unary Minus/LConn1 -- bound/RConn1 -- y contact force/LConn4
  Unary Minus/RConn1 -- x contact force/LConn5 -- y contact force/LConn5
  x contact force/LConn1 -- y contact force/LConn1 -- PS Switch/LConn1 -- Frictionless/RConn1
  PS Switch/LConn3 -- z update/RConn1

== system NUgus_IK/NUgus/left_foot/foot_fr_contact/calculate forces ==
  Frictionless : fl_lib/Physical Signals/Sources/PS Constant  constant=0
  PS Switch : fl_lib/Physical Signals/Nonlinear Operators/PS Switch  Threshold=0
      settings: SourceProductName=Simscape  SourceProductBaseCode=SS
  Unary Minus : fl_lib/Physical Signals/Functions/PS Gain  gain=-1
  x contact force : Subsystem
  y contact force : Subsystem
  x velocity : PMIOPort  Side=Left
  y velocity : PMIOPort  Port=2  Side=Left
  z position : PMIOPort  Port=3  Side=Left
  z update : PMIOPort  Port=4  Side=Left
  bound : PMIOPort  Port=5  Side=Left
  x force : PMIOPort  Port=6  Side=Right
  y force : PMIOPort  Port=7  Side=Right
  z force : PMIOPort  Port=8  Side=Right
  connections:
  x contact force/LConn2 -- x velocity/RConn1
  y contact force/LConn2 -- y velocity/RConn1
  y contact force/RConn1 -- y force/RConn1
  x contact force/RConn1 -- x force/RConn1
  PS Switch/RConn1 -- z force/RConn1
  x contact force/LConn3 -- PS Switch/LConn2 -- z position/RConn1 -- y contact force/LConn3
  x contact force/LConn4 -- Unary Minus/LConn1 -- bound/RConn1 -- y contact force/LConn4
  Unary Minus/RConn1 -- x contact force/LConn5 -- y contact force/LConn5
  x contact force/LConn1 -- y contact force/LConn1 -- PS Switch/LConn1 -- Frictionless/RConn1
  PS Switch/LConn3 -- z update/RConn1

== system NUgus_IK/NUgus/right_foot/foot_bl_contact/calculate forces ==
  Frictionless : fl_lib/Physical Signals/Sources/PS Constant  constant=0
  PS Switch : fl_lib/Physical Signals/Nonlinear Operators/PS Switch  Threshold=0
      settings: SourceProductName=Simscape  SourceProductBaseCode=SS
  Unary Minus : fl_lib/Physical Signals/Functions/PS Gain  gain=-1
  x contact force : Subsystem
  y contact force : Subsystem
  x velocity : PMIOPort  Side=Left
  y velocity : PMIOPort  Port=2  Side=Left
  z position : PMIOPort  Port=3  Side=Left
  z update : PMIOPort  Port=4  Side=Left
  bound : PMIOPort  Port=5  Side=Left
  x force : PMIOPort  Port=6  Side=Right
  y force : PMIOPort  Port=7  Side=Right
  z force : PMIOPort  Port=8  Side=Right
  connections:
  x contact force/LConn2 -- x velocity/RConn1
  y contact force/LConn2 -- y velocity/RConn1
  y contact force/RConn1 -- y force/RConn1
  x contact force/RConn1 -- x force/RConn1
  PS Switch/RConn1 -- z force/RConn1
  x contact force/LConn3 -- PS Switch/LConn2 -- z position/RConn1 -- y contact force/LConn3
  x contact force/LConn4 -- Unary Minus/LConn1 -- bound/RConn1 -- y contact force/LConn4
  Unary Minus/RConn1 -- x contact force/LConn5 -- y contact force/LConn5
  x contact force/LConn1 -- y contact force/LConn1 -- PS Switch/LConn1 -- Frictionless/RConn1
  PS Switch/LConn3 -- z update/RConn1

== system NUgus_IK/NUgus/right_foot/foot_br_contact/calculate forces ==
  Frictionless : fl_lib/Physical Signals/Sources/PS Constant  constant=0
  PS Switch : fl_lib/Physical Signals/Nonlinear Operators/PS Switch  Threshold=0
      settings: SourceProductName=Simscape  SourceProductBaseCode=SS
  Unary Minus : fl_lib/Physical Signals/Functions/PS Gain  gain=-1
  x contact force : Subsystem
  y contact force : Subsystem
  x velocity : PMIOPort  Side=Left
  y velocity : PMIOPort  Port=2  Side=Left
  z position : PMIOPort  Port=3  Side=Left
  z update : PMIOPort  Port=4  Side=Left
  bound : PMIOPort  Port=5  Side=Left
  x force : PMIOPort  Port=6  Side=Right
  y force : PMIOPort  Port=7  Side=Right
  z force : PMIOPort  Port=8  Side=Right
  connections:
  x contact force/LConn2 -- x velocity/RConn1
  y contact force/LConn2 -- y velocity/RConn1
  y contact force/RConn1 -- y force/RConn1
  x contact force/RConn1 -- x force/RConn1
  PS Switch/RConn1 -- z force/RConn1
  x contact force/LConn3 -- y contact force/LConn3 -- PS Switch/LConn2 -- z position/RConn1
  x contact force/LConn4 -- y contact force/LConn4 -- Unary Minus/LConn1 -- bound/RConn1
  x contact force/LConn5 -- y contact force/LConn5 -- Unary Minus/RConn1
  x contact force/LConn1 -- Frictionless/RConn1 -- y contact force/LConn1 -- PS Switch/LConn1
  PS Switch/LConn3 -- z update/RConn1

== system NUgus_IK/NUgus/right_foot/foot_fl_contact/calculate forces ==
  Frictionless : fl_lib/Physical Signals/Sources/PS Constant  constant=0
  PS Switch : fl_lib/Physical Signals/Nonlinear Operators/PS Switch  Threshold=0
      settings: SourceProductName=Simscape  SourceProductBaseCode=SS
  Unary Minus : fl_lib/Physical Signals/Functions/PS Gain  gain=-1
  x contact force : Subsystem
  y contact force : Subsystem
  x velocity : PMIOPort  Side=Left
  y velocity : PMIOPort  Port=2  Side=Left
  z position : PMIOPort  Port=3  Side=Left
  z update : PMIOPort  Port=4  Side=Left
  bound : PMIOPort  Port=5  Side=Left
  x force : PMIOPort  Port=6  Side=Right
  y force : PMIOPort  Port=7  Side=Right
  z force : PMIOPort  Port=8  Side=Right
  connections:
  x contact force/LConn2 -- x velocity/RConn1
  y contact force/LConn2 -- y velocity/RConn1
  y contact force/RConn1 -- y force/RConn1
  x contact force/RConn1 -- x force/RConn1
  PS Switch/RConn1 -- z force/RConn1
  x contact force/LConn3 -- PS Switch/LConn2 -- z position/RConn1 -- y contact force/LConn3
  x contact force/LConn4 -- Unary Minus/LConn1 -- bound/RConn1 -- y contact force/LConn4
  Unary Minus/RConn1 -- x contact force/LConn5 -- y contact force/LConn5
  x contact force/LConn1 -- y contact force/LConn1 -- PS Switch/LConn1 -- Frictionless/RConn1
  PS Switch/LConn3 -- z update/RConn1

== system NUgus_IK/NUgus/right_foot/foot_fr_contact/calculate forces ==
  Frictionless : fl_lib/Physical Signals/Sources/PS Constant  constant=0
  PS Switch : fl_lib/Physical Signals/Nonlinear Operators/PS Switch  Threshold=0
      settings: SourceProductName=Simscape  SourceProductBaseCode=SS
  Unary Minus : fl_lib/Physical Signals/Functions/PS Gain  gain=-1
  x contact force : Subsystem
  y contact force : Subsystem
  x velocity : PMIOPort  Side=Left
  y velocity : PMIOPort  Port=2  Side=Left
  z position : PMIOPort  Port=3  Side=Left
  z update : PMIOPort  Port=4  Side=Left
  bound : PMIOPort  Port=5  Side=Left
  x force : PMIOPort  Port=6  Side=Right
  y force : PMIOPort  Port=7  Side=Right
  z force : PMIOPort  Port=8  Side=Right
  connections:
  x contact force/LConn2 -- x velocity/RConn1
  y contact force/LConn2 -- y velocity/RConn1
  y contact force/RConn1 -- y force/RConn1
  x contact force/RConn1 -- x force/RConn1
  PS Switch/RConn1 -- z force/RConn1
  x contact force/LConn3 -- PS Switch/LConn2 -- z position/RConn1 -- y contact force/LConn3
  x contact force/LConn4 -- Unary Minus/LConn1 -- bound/RConn1 -- y contact force/LConn4
  Unary Minus/RConn1 -- x contact force/LConn5 -- y contact force/LConn5
  x contact force/LConn1 -- y contact force/LConn1 -- PS Switch/LConn1 -- Frictionless/RConn1
  PS Switch/LConn3 -- z update/RConn1

== system NUgus_IK/NUgus/torso/IMU/Convert Acc ==
  PS-Simulink Converter : nesl_utility/PS-Simulink Converter  PhysicalDomain=network_engine_domain  SubClassName=ps_output  LeftPortType=input  RightPortType=output  PseudoPeriodic=off  Frequencies=[]  Unit=m/s^2  AffineConversion=off
  PS-Simulink Converter1 : nesl_utility/PS-Simulink Converter  PhysicalDomain=network_engine_domain  SubClassName=ps_output  LeftPortType=input  RightPortType=output  PseudoPeriodic=off  Frequencies=[]  Unit=m/s^2  AffineConversion=off
  PS-Simulink Converter2 : nesl_utility/PS-Simulink Converter  PhysicalDomain=network_engine_domain  SubClassName=ps_output  LeftPortType=input  RightPortType=output  PseudoPeriodic=off  Frequencies=[]  Unit=m/s^2  AffineConversion=off
  PS-Simulink Converter3 : nesl_utility/PS-Simulink Converter  PhysicalDomain=network_engine_domain  SubClassName=ps_output  LeftPortType=input  RightPortType=output  PseudoPeriodic=off  Frequencies=[]  Unit=1  AffineConversion=off
  Ha : PMIOPort  Side=Left
  x : PMIOPort  Port=2  Side=Left
  y : PMIOPort  Port=3  Side=Left
  z : PMIOPort  Port=4  Side=Left
  Htw : Outport
  ax : Outport  Port=2
  ay : Outport  Port=3
  az : Outport  Port=4
  wires:
  PS-Simulink Converter2/1 -> az/1
  PS-Simulink Converter1/1 -> ay/1
  PS-Simulink Converter/1 -> ax/1
  PS-Simulink Converter3/1 -> Htw/1
  connections:
  PS-Simulink Converter2/LConn1 -- z/RConn1
  PS-Simulink Converter/LConn1 -- x/RConn1
  PS-Simulink Converter1/LConn1 -- y/RConn1
  Ha/RConn1 -- PS-Simulink Converter3/LConn1

== system NUgus_IK/NUgus/torso/IMU/Convert Gyro ==
  PS-Simulink Converter : nesl_utility/PS-Simulink Converter  PhysicalDomain=network_engine_domain  SubClassName=ps_output  LeftPortType=input  RightPortType=output  PseudoPeriodic=off  Frequencies=[]  Unit=rad/s  AffineConversion=off
  PS-Simulink Converter1 : nesl_utility/PS-Simulink Converter  PhysicalDomain=network_engine_domain  SubClassName=ps_output  LeftPortType=input  RightPortType=output  PseudoPeriodic=off  Frequencies=[]  Unit=rad/s  AffineConversion=off
  PS-Simulink Converter2 : nesl_utility/PS-Simulink Converter  PhysicalDomain=network_engine_domain  SubClassName=ps_output  LeftPortType=input  RightPortType=output  PseudoPeriodic=off  Frequencies=[]  Unit=rad/s  AffineConversion=off
  x : PMIOPort  Side=Left
  y : PMIOPort  Port=2  Side=Left
  z : PMIOPort  Port=3  Side=Left
  wx : Outport
  wy : Outport  Port=2
  wz : Outport  Port=3
  wires:
  PS-Simulink Converter2/1 -> wz/1
  PS-Simulink Converter1/1 -> wy/1
  PS-Simulink Converter/1 -> wx/1
  connections:
  PS-Simulink Converter2/LConn1 -- z/RConn1
  PS-Simulink Converter/LConn1 -- x/RConn1
  PS-Simulink Converter1/LConn1 -- y/RConn1

== system NUgus_IK/NUgus/torso/IMU/Saturate Acc ==
  Hta : Inport
  Acc : Inport  Port=2
  Acc Saturation : Saturate  UpperLimit=1023  LowerLimit=0
  Add : Sum  Inputs=+++
  Constant : Constant  Value=CM740_acc_bias
  Constant1 : Constant  Value=[0 0 9.80743]
  Gain1 : Gain  Gain=CM740_acc_gain  OutDataTypeStr=int16
  Matrix Multiply : Product  Multiplication=Matrix(*)
  Transpose : Math  Operator=transpose  SaturateOnIntegerOverflow=on
  alpha : Outport
  wires:
  Acc/1 -> Add/3
  Add/1 -> Gain1/1
  Acc Saturation/1 -> alpha/1
  Matrix Multiply/1 -> Add/1
  Gain1/1 -> Acc Saturation/1
  Constant/1 -> Add/2
  Transpose/1 -> Matrix Multiply/1
  Hta/1 -> Transpose/1
  Constant1/1 -> Matrix Multiply/2

== system NUgus_IK/NUgus/torso/IMU/Saturate Gyro ==
  w : Inport
  Add1 : Sum
  Constant1 : Constant  Value=CM740_gyro_bias
  Gain : Gain  Gain=CM740_gyro_gain  OutDataTypeStr=int16
  Gyro Saturation : Saturate  UpperLimit=1023  LowerLimit=0
  omega : Outport
  wires:
  Constant1/1 -> Add1/2
  Gyro Saturation/1 -> omega/1
  Add1/1 -> Gain/1
  Gain/1 -> Gyro Saturation/1
  w/1 -> Add1/1

== system NUgus_IK/NUgus/left_foot/foot_bl_contact/calculate forces/x contact force ==
  PS Max1 : fl_lib/Physical Signals/Nonlinear Operators/PS Max
      settings: SourceProductName=Simscape  SourceProductBaseCode=SS
  PS Min1 : fl_lib/Physical Signals/Nonlinear Operators/PS Min
      settings: SourceProductName=Simscape  SourceProductBaseCode=SS
  PS Switch : fl_lib/Physical Signals/Nonlinear Operators/PS Switch  Threshold=0
      settings: SourceProductName=Simscape  SourceProductBaseCode=SS
  frictionless : PMIOPort  Side=Left
  force : PMIOPort  Port=2  Side=Right
  velocity : PMIOPort  Port=3  Side=Left
  z position : PMIOPort  Port=4  Side=Left
  upper_bound : PMIOPort  Port=5  Side=Left
  lower_bound : PMIOPort  Port=6  Side=Left
  connections:
  PS Max1/LConn2 -- lower_bound/RConn1
  PS Max1/LConn1 -- PS Min1/RConn1
  PS Switch/LConn3 -- PS Max1/RConn1
  PS Min1/LConn1 -- velocity/RConn1
  PS Switch/LConn2 -- z position/RConn1
  PS Switch/LConn1 -- frictionless/RConn1
  PS Switch/RConn1 -- force/RConn1
  upper_bound/RConn1 -- PS Min1/LConn2

== system NUgus_IK/NUgus/left_foot/foot_bl_contact/calculate forces/y contact force ==
  PS Max1 : fl_lib/Physical Signals/Nonlinear Operators/PS Max
      settings: SourceProductName=Simscape  SourceProductBaseCode=SS
  PS Min1 : fl_lib/Physical Signals/Nonlinear Operators/PS Min
      settings: SourceProductName=Simscape  SourceProductBaseCode=SS
  PS Switch : fl_lib/Physical Signals/Nonlinear Operators/PS Switch  Threshold=0
      settings: SourceProductName=Simscape  SourceProductBaseCode=SS
  frictionless : PMIOPort  Side=Left
  force : PMIOPort  Port=2  Side=Right
  velocity : PMIOPort  Port=3  Side=Left
  z position : PMIOPort  Port=4  Side=Left
  upper_bound : PMIOPort  Port=5  Side=Left
  lower_bound : PMIOPort  Port=6  Side=Left
  connections:
  PS Max1/LConn2 -- lower_bound/RConn1
  PS Max1/LConn1 -- PS Min1/RConn1
  PS Switch/LConn3 -- PS Max1/RConn1
  PS Min1/LConn1 -- velocity/RConn1
  PS Switch/LConn2 -- z position/RConn1
  PS Switch/LConn1 -- frictionless/RConn1
  PS Switch/RConn1 -- force/RConn1
  upper_bound/RConn1 -- PS Min1/LConn2

== system NUgus_IK/NUgus/left_foot/foot_br_contact/calculate forces/x contact force ==
  PS Max1 : fl_lib/Physical Signals/Nonlinear Operators/PS Max
      settings: SourceProductName=Simscape  SourceProductBaseCode=SS
  PS Min1 : fl_lib/Physical Signals/Nonlinear Operators/PS Min
      settings: SourceProductName=Simscape  SourceProductBaseCode=SS
  PS Switch : fl_lib/Physical Signals/Nonlinear Operators/PS Switch  Threshold=0
      settings: SourceProductName=Simscape  SourceProductBaseCode=SS
  frictionless : PMIOPort  Side=Left
  force : PMIOPort  Port=2  Side=Right
  velocity : PMIOPort  Port=3  Side=Left
  z position : PMIOPort  Port=4  Side=Left
  upper_bound : PMIOPort  Port=5  Side=Left
  lower_bound : PMIOPort  Port=6  Side=Left
  connections:
  PS Max1/LConn2 -- lower_bound/RConn1
  PS Max1/LConn1 -- PS Min1/RConn1
  PS Switch/LConn3 -- PS Max1/RConn1
  PS Min1/LConn1 -- velocity/RConn1
  PS Switch/LConn2 -- z position/RConn1
  PS Switch/LConn1 -- frictionless/RConn1
  PS Switch/RConn1 -- force/RConn1
  upper_bound/RConn1 -- PS Min1/LConn2

== system NUgus_IK/NUgus/left_foot/foot_br_contact/calculate forces/y contact force ==
  PS Max1 : fl_lib/Physical Signals/Nonlinear Operators/PS Max
      settings: SourceProductName=Simscape  SourceProductBaseCode=SS
  PS Min1 : fl_lib/Physical Signals/Nonlinear Operators/PS Min
      settings: SourceProductName=Simscape  SourceProductBaseCode=SS
  PS Switch : fl_lib/Physical Signals/Nonlinear Operators/PS Switch  Threshold=0
      settings: SourceProductName=Simscape  SourceProductBaseCode=SS
  frictionless : PMIOPort  Side=Left
  force : PMIOPort  Port=2  Side=Right
  velocity : PMIOPort  Port=3  Side=Left
  z position : PMIOPort  Port=4  Side=Left
  upper_bound : PMIOPort  Port=5  Side=Left
  lower_bound : PMIOPort  Port=6  Side=Left
  connections:
  PS Max1/LConn2 -- lower_bound/RConn1
  PS Max1/LConn1 -- PS Min1/RConn1
  PS Switch/LConn3 -- PS Max1/RConn1
  PS Min1/LConn1 -- velocity/RConn1
  PS Switch/LConn2 -- z position/RConn1
  PS Switch/LConn1 -- frictionless/RConn1
  PS Switch/RConn1 -- force/RConn1
  upper_bound/RConn1 -- PS Min1/LConn2
